simulink library "smdoc_simple_rigid_bodies"  (R2021b)
settings: Solver=ode45  StartTime=0.0  StopTime=10.0  RelTol=1e-3  EnableMultiTasking=on
libraries: sm_lib x5
settings Model: Creator=The MathWorks, Inc.  LastModifiedBy=The MathWorks, Inc.
settings SolverCC: AlgebraicLoopSolver=TrustRegion
settings DataIOCC: LimitDataPoints=on  SaveFormat=Array  ReturnWorkspaceOutputs=off
settings OptimizationCC: LifeSpan=inf
settings DebuggingCC: UnderspecifiedInitializationDetection=Classic  MergeDetectMultiDrivingBlocksExec=none  SolverPrmCheckMsg=warning  SFUnexpectedBacktrackingDiag=warning  SFNoUnconditionalDefaultTransitionDiag=warning  SFExecutionAtInitializationDiag=none  SFMachineParentedDataDiag=warning  ArithmeticOperatorsInVariantConditions=warning
settings HardwareCC: ProdBitPerPointer=32  ProdBitPerSizeT=32  ProdBitPerPtrDiffT=32  ProdLargestAtomicFloat=None  ProdIntDivRoundTo=Undefined  ProdEndianess=Unspecified  ProdWordSize=32  ProdHWDeviceType=32-bit Generic
settings ModelReferenceCC: PropagateSignalLabelsOutOfModel=off
settings SFSimCC: SimUseLocalCustomCode=off  SimGenImportedTypeDefs=on  CustomCodeUndefinedFunction=UseInterfaceOnly
settings RTWCC: RTWUseLocalCustomCode=off
settings CodeAppCC: StateflowObjectComments=on
settings GRTTargetCC: TargetLangStandard=C89/C90 (ANSI)
settings ConfigComp: CovMetricSettings=dw  CovSaveCumulativeToWorkspaceVar=on  CovSaveSingleToWorkspaceVar=on  CovExternalEMLEnable=off

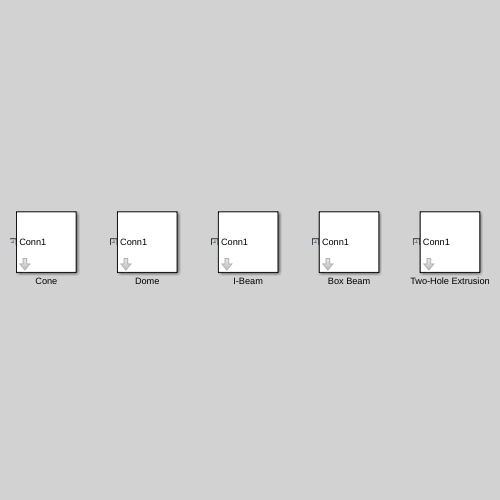
[thumbnail: Simulink's stored preview of the top-level diagram]
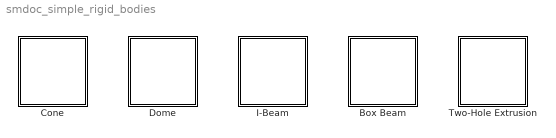
== system smdoc_simple_rigid_bodies ==
  Box Beam : Subsystem  mask{L=10, H=4, W=2, T=0.2, RGB=[0.85 0.45 0]}
      mask prompts: L "Length"; H "Height"; W "Width"; T "Thickness"; RGB "Color"
      mask init:
      | D1 = W/2-T;
      | D2 = H/2-T;
      | OuterCS = [-W/2,-H/2; W/2,-H/2; W/2,H/2; ...
      | -W/2,H/2; -W/2,-H/2];
      | InnerCS = [-D1,-D2; -D1,D2; D1,D2; D1 -D2; -D1,-D2];
      | CS = [OuterCS; InnerCS];
  Cone : Subsystem  mask{R=1, H=2, T=0.1, RGB=[0.85 0.45 0]}
      mask prompts: R "Base Radius"; H "Cone Height"; T "Wall Thickness"; RGB "Color"
      mask init:
      | Alpha = atan(R/H);
      | CS = [0 0; R H; R-T/cos(Alpha) H; 0 T/sin(Alpha)];
  Dome : Subsystem  mask{R=1, T=0.1, RGB=[0.85 0.45 0]}
      mask prompts: R "Base Radius"; T "Wall Thickness"; RGB "Color"
      mask init:
      | % Circular dome outer coordinates:
      | Alpha = (0:0.01:pi/2)';
      | OuterCS = R*[cos(Alpha), sin(Alpha)];
      | 
      | % Circular dome inner coordinates:
      | Beta = (pi/2:-0.01:0)';
      | InnerCS = (R-T)*[cos(Beta), sin(Beta)];
      | 
      | CS = [OuterCS; InnerCS];
  I-Beam : Subsystem  mask{L=10, H=4, W=2, T=0.2, RGB=[0.85 0.45 0]}
      mask prompts: L "Length"; H "Height"; W "Width"; T "Thickness"; RGB "Color"
      mask init:
      | D = H/2-T;
      | HalfCS = [W/2, -H/2; W/2, -D; T/2, -D;
      | T/2, D; W/2, D; W/2, H/2];
      | CS = [HalfCS; -HalfCS];
  Two-Hole Extrusion : Subsystem  mask{L=1, Ro=10, Ri=3, Rho=2700, RGB=[0.85 0.45 0]}
      mask prompts: L "Extrusion Length (cm)"; Ro "Extrusion Outer Radius (cm)"; Ri "Hole Radius (cm)"; Rho "Mass Density (kg/m^3)"; RGB "Color [R G B]"
      mask init:
      | % External Cross-Section
      | Theta = (0:0.001:2*pi)';
      | CS = [Ro*cos(Theta), Ro*sin(Theta)];
      | 
      | % Hole Cross-Sections
      | Theta = (0:-0.001:-pi)';
      | Alpha = (pi:-0.001:0)';
      | 
      | A = [Ro/2 + Ri*cos(Theta), Ri*sin(Theta)];
      | B = [-Ro/2 + Ri*cos(Theta), Ri*sin(Theta)];
      | C = [-Ro/2 + Ri*cos(Alpha), Ri*sin(Alpha)];
      | D = [Ro/2 + Ri*cos(Alpha), Ri*sin(Alpha)];
      | 
      | CS = [CS; A; B; C; D];

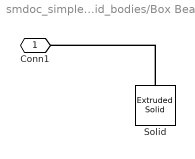
== system smdoc_simple_rigid_bodies/Box Beam ==
  Solid : sm_lib/Body Elements/Extruded Solid  GraphicAmbientColor=[0.15 0.15 0.15 1.0]  BasedOnType=Density  CenterOfMass=[0 0 0]  CenterOfMassUnits=m  GraphicDiffuseColor=RGB  ExportConvexHullGeometry=off  ExtrusionCrossSection=CS  ExtrusionCrossSectionUnits=cm  Density=1000  DensityUnits=kg/(m^3)  DoExposeReferenceFrame=on  GraphicEmissiveColor=[0.0 0.0 0.0 1.0]  ExportEntireGeometry=off  ExtrusionLength=L  ExtrusionLengthUnits=cm  ExtrusionType=General  SerializedFrames=<Frames/>  MarkerShape=Sphere  MarkerSize=10  GraphicType=FromGeometry  InertiaType=CalculateFromGeometry  Mass=1  MassUnits=kg  MomentsOfInertia=[1 1 1]  MomentsOfInertiaUnits=kg*m^2  PolygonNumSides=3  GraphicOpacity=1.0  PolygonOuterRadius=1  PolygonOuterRadiusUnits=m  ProductsOfInertia=[0 0 0]  ProductsOfInertiaUnits=kg*m^2  GraphicShininess=75  GraphicSpecularColor=[0.5 0.5 0.5 1.0]  GraphicVisPropType=SimpleVisualProperties
  Conn1 : PMIOPort  Side=Left
  connections:
  Solid/RConn1 -- Conn1/RConn1

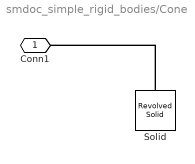
== system smdoc_simple_rigid_bodies/Cone ==
  Solid : sm_lib/Body Elements/Revolved Solid  GraphicAmbientColor=[0.15 0.15 0.15 1.0]  BasedOnType=Density  CenterOfMass=[0 0 0]  CenterOfMassUnits=m  GraphicDiffuseColor=RGB  ExportConvexHullGeometry=off  Density=1000  DensityUnits=kg/(m^3)  DoExposeReferenceFrame=on  GraphicEmissiveColor=[0.0 0.0 0.0 1.0]  ExportEntireGeometry=off  SerializedFrames=<Frames/>  MarkerShape=Sphere  MarkerSize=10  GraphicType=FromGeometry  InertiaType=CalculateFromGeometry  Mass=1  MassUnits=kg  MomentsOfInertia=[1 1 1]  MomentsOfInertiaUnits=kg*m^2  GraphicOpacity=1.0  ProductsOfInertia=[0 0 0]  ProductsOfInertiaUnits=kg*m^2  RevolutionCrossSection=CS  RevolutionCrossSectionUnits=cm  RevolutionAngle=180  RevolutionAngleUnits=deg  RevolutionExtent=Full  GraphicShininess=75  GraphicSpecularColor=[0.5 0.5 0.5 1.0]  GraphicVisPropType=SimpleVisualProperties
  Conn1 : PMIOPort  Side=Left
  connections:
  Solid/RConn1 -- Conn1/RConn1

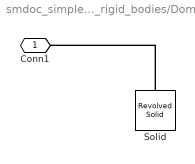
== system smdoc_simple_rigid_bodies/Dome ==
  Solid : sm_lib/Body Elements/Revolved Solid  GraphicAmbientColor=[0.15 0.15 0.15 1.0]  BasedOnType=Density  CenterOfMass=[0 0 0]  CenterOfMassUnits=m  GraphicDiffuseColor=RGB  ExportConvexHullGeometry=off  Density=1000  DensityUnits=kg/(m^3)  DoExposeReferenceFrame=on  GraphicEmissiveColor=[0.0 0.0 0.0 1.0]  ExportEntireGeometry=off  SerializedFrames=<Frames/>  MarkerShape=Sphere  MarkerSize=10  GraphicType=FromGeometry  InertiaType=CalculateFromGeometry  Mass=1  MassUnits=kg  MomentsOfInertia=[1 1 1]  MomentsOfInertiaUnits=kg*m^2  GraphicOpacity=1.0  ProductsOfInertia=[0 0 0]  ProductsOfInertiaUnits=kg*m^2  RevolutionCrossSection=CS  RevolutionCrossSectionUnits=cm  RevolutionAngle=180  RevolutionAngleUnits=deg  RevolutionExtent=Full  GraphicShininess=75  GraphicSpecularColor=[0.5 0.5 0.5 1.0]  GraphicVisPropType=SimpleVisualProperties
  Conn1 : PMIOPort  Side=Left
  connections:
  Solid/RConn1 -- Conn1/RConn1

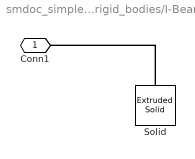
== system smdoc_simple_rigid_bodies/I-Beam ==
  Solid : sm_lib/Body Elements/Extruded Solid  GraphicAmbientColor=[0.15 0.15 0.15 1.0]  BasedOnType=Density  CenterOfMass=[0 0 0]  CenterOfMassUnits=m  GraphicDiffuseColor=RGB  ExportConvexHullGeometry=off  ExtrusionCrossSection=CS  ExtrusionCrossSectionUnits=cm  Density=1000  DensityUnits=kg/(m^3)  DoExposeReferenceFrame=on  GraphicEmissiveColor=[0.0 0.0 0.0 1.0]  ExportEntireGeometry=off  ExtrusionLength=L  ExtrusionLengthUnits=cm  ExtrusionType=General  SerializedFrames=<Frames/>  MarkerShape=Sphere  MarkerSize=10  GraphicType=FromGeometry  InertiaType=CalculateFromGeometry  Mass=1  MassUnits=kg  MomentsOfInertia=[1 1 1]  MomentsOfInertiaUnits=kg*m^2  PolygonNumSides=3  GraphicOpacity=1.0  PolygonOuterRadius=1  PolygonOuterRadiusUnits=m  ProductsOfInertia=[0 0 0]  ProductsOfInertiaUnits=kg*m^2  GraphicShininess=75  GraphicSpecularColor=[0.5 0.5 0.5 1.0]  GraphicVisPropType=SimpleVisualProperties
  Conn1 : PMIOPort  Side=Left
  connections:
  Solid/RConn1 -- Conn1/RConn1

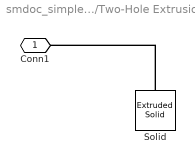
== system smdoc_simple_rigid_bodies/Two-Hole Extrusion ==
  Solid : sm_lib/Body Elements/Extruded Solid  GraphicAmbientColor=[0.15 0.15 0.15 1.0]  BasedOnType=Density  CenterOfMass=[0 0 0]  CenterOfMassUnits=m  GraphicDiffuseColor=RGB  ExportConvexHullGeometry=off  ExtrusionCrossSection=CS  ExtrusionCrossSectionUnits=cm  Density=Rho  DensityUnits=kg/(m^3)  DoExposeReferenceFrame=on  GraphicEmissiveColor=[0.0 0.0 0.0 1.0]  ExportEntireGeometry=off  ExtrusionLength=L  ExtrusionLengthUnits=cm  ExtrusionType=General  SerializedFrames=<Frames/>  MarkerShape=Sphere  MarkerSize=10  GraphicType=FromGeometry  InertiaType=CalculateFromGeometry  Mass=1  MassUnits=kg  MomentsOfInertia=[1 1 1]  MomentsOfInertiaUnits=kg*m^2  PolygonNumSides=3  GraphicOpacity=1.0  PolygonOuterRadius=1  PolygonOuterRadiusUnits=m  ProductsOfInertia=[0 0 0]  ProductsOfInertiaUnits=kg*m^2  GraphicShininess=75  GraphicSpecularColor=[0.5 0.5 0.5 1.0]  GraphicVisPropType=SimpleVisualProperties
  Conn1 : PMIOPort  Side=Left
  connections:
  Solid/RConn1 -- Conn1/RConn1
